simulink model "new24a"  (R2024a)
settings: Solver=FixedStepAuto  StartTime=0  StopTime=3  FixedStep=1e-6  RelTol=1e-3
InitFcn:
  | vdc=400
  | fsw=10000
  | Ld=0.393e-3
  | Lq=0.617e-3
  | R=0.0325
  | p=4
  | PM_flux=0.059
  | J=0.037
  | B=0.005
  | 
  | % Vehicle Model
  | Gr=1/5;                    %Gear Ratio
  | Trd=.508/2;                %Tire Radius
  | Drag= .25  ;               % Aro Dynamic Drag
  | Af= 2.23   ;               %Fontal Area
  | row= 1.225   ;             % Air Resistance
  | %Vm=260+140 ;              %Vehicle Weight
  | Vm=100;
  | Vw= Vm*9.81    ;           % Vehicle weight
  | Crr= .013  ;               %Rolling Coefficient
libraries: spsControlledVoltageSourceLib x1, slpidlib x1, spsPermanentMagnetSynchronousMachineLib x1, rllib x1, spsUniversalBridgeLib x1, spsabctodq0Lib x1, sps_lib x1
settings Model: Creator=lyche  LastModifiedBy=Saswata Mahato
settings SolverCC: ZeroCrossAlgorithm=Adaptive  AlgebraicLoopSolver=TrustRegion
settings DataIOCC: ReturnWorkspaceOutputs=off
settings OptimizationCC: ReuseModelBlockBuffer=off
settings DebuggingCC: MaxConsecutiveZCsMsg=none  UnconnectedInputMsg=warning  UnconnectedOutputMsg=warning  UnconnectedLineMsg=warning  ArithmeticOperatorsInVariantConditions=warning
settings ModelReferenceCC: EnableRefExpFcnMdlSchedulingChecks=on
settings SFSimCC: SimUseLocalCustomCode=off  CustomCodeUndefinedFunction=UseInterfaceOnly
settings RTWCC: RTWUseLocalCustomCode=off  GPUComputeCapability=3.5
settings CodeAppCC: StateflowObjectComments=on
settings SimscapeCC: SimscapeNormalizeSystem=off

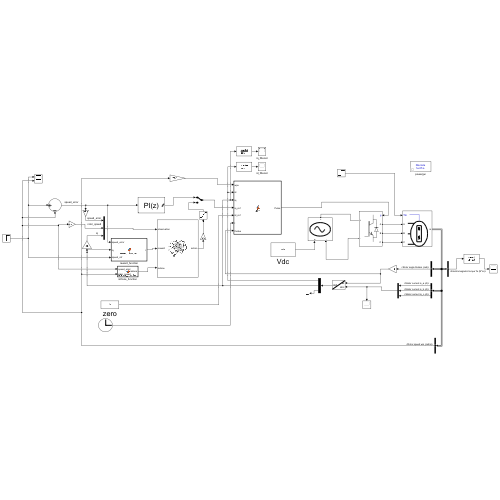
[thumbnail: Simulink's stored preview of the top-level diagram]
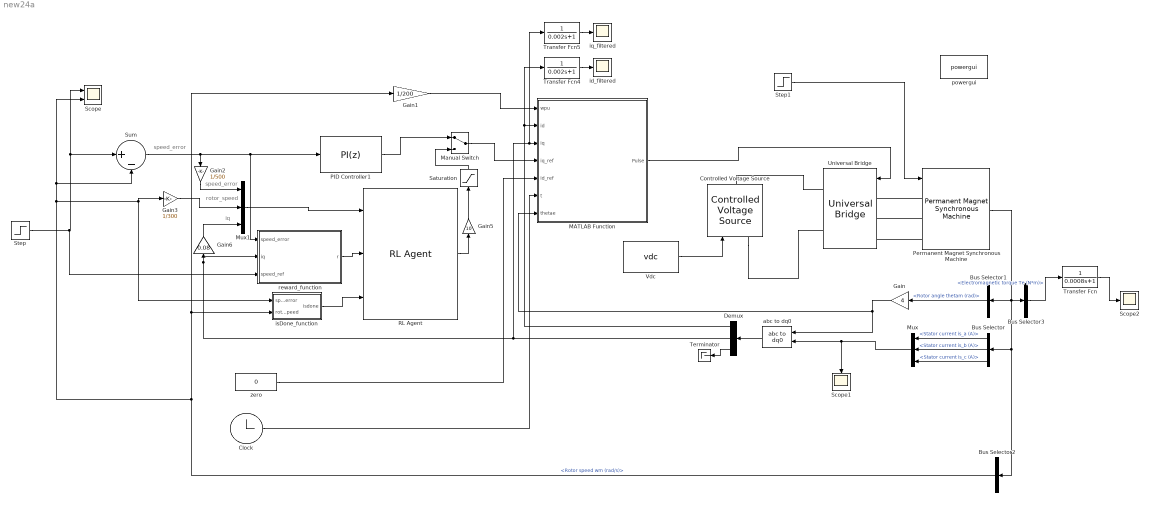
== system new24a ==
  note: iq
  note: rotor_speed
  note: speed_error
  note: speed_error
  Bus Selector : BusSelector  OutputSignals=Stator current is_a (A),Stator current is_b (A),Stator current is_c (A)
  Bus Selector1 : BusSelector  OutputSignals=Rotor angle thetam (rad)
  Bus Selector2 : BusSelector  OutputSignals=Rotor speed wm (rad/s)
  Bus Selector3 : BusSelector  OutputSignals=Electromagnetic torque Te (N*m)
  Clock : Clock
  Controlled Voltage Source : spsControlledVoltageSourceLib/Controlled Voltage Source  Initialize=off  Source_Type=AC  Amplitude=0  Phase=0  Frequency=0  Measurements=None
  Demux : Demux  Outputs=3
  Gain : Gain  Gain=4
  Gain1 : Gain  Gain=1/200
  Gain2 : Gain  Gain=1/500
  Gain3 : Gain  Gain=1/300
  Gain5 : Gain  Gain=10
  Gain6 : Gain  Gain=0.08
  MATLAB Function : MATLAB Function  TreatAsAtomicUnit=on
  Manual Switch : ManualSwitch
  Mux : Mux  Inputs=3
  Mux1 : Mux  Inputs=3
  PID Controller1 : slpidlib/PID Controller  Controller=PI  Form=Parallel  TimeDomain=Discrete-time  UseExternalTs=off  SampleTime=-1  IntegratorMethod=Forward Euler  FilterMethod=Forward Euler  ControllerParametersSource=internal  P=65.672  I=8.8746  UseKiTs=off  D=0  UseExternalDerivativeSource=off  N=100  UseFilter=on  TunerSelectOption=Transfer Function Based (PID Tuner App)  InitialConditionSource=internal  InitialConditionForIntegrator=0  InitialConditionForFilter=0  DifferentiatorICPrevScaledInput=0  ExternalReset=none  TrackingMode=off  Kt=1  LimitOutput=on  SatLimitsSource=internal  UpperSaturationLimit=500  LowerSaturationLimit=-500  LinearizeAsGain=off  AntiWindupMode=none  Kb=1  LimitIntegrator=off  UpperIntegratorSaturationLimit=inf  LowerIntegratorSaturationLimit=-inf  POutMin=[]  POutMax=[]  IOutMin=[]  IOutMax=[]  DOutMin=[]  DOutMax=[]  NOutMin=[]  NOutMax=[]  SumOutMin=[]  SumOutMax=[]  SaturationOutMin=[]  SaturationOutMax=[]  PParamMin=[]  PParamMax=[]  IParamMin=[]  IParamMax=[]  DParamMin=[]  DParamMax=[]  NParamMin=[]  NParamMax=[]  KbParamMin=[]  KbParamMax=[]  KtParamMin=[]  KtParamMax=[]  KbOutMin=[]  KbOutMax=[]  KtOutMin=[]  KtOutMax=[]  IntegratorOutMin=[]  IntegratorOutMax=[]  FilterOutMin=[]  FilterOutMax=[]  SumI1OutMin=[]  SumI1OutMax=[]  SumI2OutMin=[]  SumI2OutMax=[]  SumI3OutMin=[]  SumI3OutMax=[]  SumI4OutMin=[]  SumI4OutMax=[]  SumDOutMin=[]  SumDOutMax=[]  DifferentiatorOutMin=[]  DifferentiatorOutMax=[]  FilterDiffOutCoefMin=[]  FilterDiffOutCoefMax=[]  ReciprocalOutMin=[]  ReciprocalOutMax=[]  SumDenOutMin=[]  SumDenOutMax=[]  SumNumOutMin=[]  SumNumOutMax=[]  DivideOutMin=[]  DivideOutMax=[]  UdiffTsProdOutMin=[]  UdiffTsProdOutMax=[]  NTsProdOutMin=[]  NTsProdOutMax=[]  UintegralTsProdOutMin=[]  UintegralTsProdOutMax=[]  UngainTsProdOutMin=[]  UngainTsProdOutMax=[]  ClampingZeroOutDataTypeStr=Inherit: Inherit via back propagation  ClampingZeroOutMin=[]  ClampingZeroOutMax=[]  FilterDenConstantOutDataTypeStr=Inherit: Inherit via back propagation  FilterDenConstantOutMin=[]  FilterDenConstantOutMax=[]  PCopyOutDataTypeStr=Inherit: Inherit via back propagation  PCopyOutMin=[]  PCopyOutMax=[]  NCopyOutDataTypeStr=Inherit: Inherit via back propagation  NCopyOutMin=[]  NCopyOutMax=[]  IntegratorContinuousStateAttributes=''  IntegratorStateMustResolveToSignalObject=off  IntegratorRTWStateStorageClass=Auto  FilterContinuousStateAttributes=''  FilterStateMustResolveToSignalObject=off  FilterRTWStateStorageClass=Auto  ParallelPVariant=InternalParameters  IdealPVariant=Disabled  IVariant=InternalParameters  DVariant=Disabled  IntegratorVariant=Discrete  SatVariant=Enabled  AWVariant=Passthrough  PCopyVariant=Disabled  TRVariant=Disabled  FdbkBlocksVariant=Forward  IdealPFdbkVariant=Disabled  SatFdbkVariant=Disabled  DerivativeFilterVariant=Disabled  NVariant=Disabled  NCopyVariant=Disabled_SignalSpec  FilterICVariant=Disabled  IntegratorICVariant=InternalICs  ExternalResetVariant=Disabled  TRSumVariant=Passthrough  SumFdbkVariant=Disabled  SumVariant=Sum_PI  TsampFilterVariant=InternalTs  TsampNgainVariant=Passthrough  TsampIntegralVariant=Disabled_SignalSpec  ExternalSaturationOutDataTypeStr=Inherit: Same as second input  DerivativeSourceVariant=Disabled
  Permanent Magnet Synchronous Machine : spsPermanentMagnetSynchronousMachineLib/Permanent Magnet Synchronous Machine  NbPhases=3  FluxDistribution=Sinusoidal  RotorType=Salient-pole  MechanicalLoad=Torque Tm  PresetModel=No  ShowDetailedParameters=on  MeasurementBus=off  Resistance=0.0325  Inductance=8.5e-3  dqInductances=[0.393e-3,0.617e-3]  La=0.000395  MachineConstant=Flux linkage established by magnets (V.s)  Flux=0.059  VoltageCst=42.8057  TorqueCst=0.354  Flat=120  Mechanical=[0.037 0.005 4 0]  PolePairs=4  InitialConditions=[0,0, 0,0]  InitialConditions5ph=[0 0 0 0 0 0]  RefAngle=90 degrees behind phase A axis (modified Park)  IterativeDiscreteModel=Trapezoidal non iterative  TsBlock=-1  TsPowergui=0
  RL Agent : rllib/RL Agent  Agent=agent  ExternalActionAsInput=off  ProvideLastAction=off  ProvideCumRwd=off  TreatAsDirectFeedthrough=on  UseStrictObservationDataTypes=off
  Saturation : Saturate  UpperLimit=10  LowerLimit=-10
  Scope : Scope  NumInputPorts=2
  Scope1 : Scope
  Scope2 : Scope
  Step : Step  Time=0.5  Before=100  After=120  SampleTime=0
  Step1 : Step  Time=0.5  Before=20  After=70  SampleTime=0
  Sum : Sum  Inputs=|+-
  Terminator : Terminator
  Transfer Fcn : TransferFcn  Denominator=[0.0008 1]
  Transfer Fcn4 : TransferFcn  Denominator=[0.002 1]
  Transfer Fcn5 : TransferFcn  Denominator=[0.002 1]
  Universal Bridge : spsUniversalBridgeLib/Universal Bridge  Arms=3  SnubberResistance=1e5  SnubberCapacitance=inf  Device=IGBT / Diodes  Ron=1e-3  Lon=0  ForwardVoltages="[  0  0  ]"  ForwardVoltage=0  GTOparameters=[ 10e-6 , 20e-6 ]  IGBTparameters=[ 1e-6 , 2e-6 ]  Measurements=None  Measurements_2=None  converterType=Rectifier
  Vdc : Constant  Value=vdc
  abc to dq0 : spsabctodq0Lib/abc to dq0  Alignment=90 degrees behind phase A axis
  id_filtered : Scope
  iq_filtered : Scope
  "isDone_function " : MATLAB Function  TreatAsAtomicUnit=on
  powergui : sps_lib/powergui  Priority=1  SimulationMode=Discrete  SampleTime=10e-6  frequency=60  Iterations=50  frequencyindice=0  Pbase=100e6  ErrMax=1e-4  UnitsV=kV  UnitsW=MW  buscounter=0  FunctionMessages=off  echomessages=off  EnableUseOfTLC=off  CurrentSourceSwitches=off  DisableSnubberDevices=off  DisableRonSwitches=off  DisableVfSwitches=off  DisplayEquations=off  AutomaticDiscreteSolvers=off  SolverType=Tustin/Backward Euler (TBE)  Interpol=off  ExternalGateDelay=off  methode=off  Ts=100  x0status=blocks  SPID=on  SwTol=0  HookPort=off  NonlinearTolerance=1e-4  nMaxIteration=100  ContinueOnMaxIteration=off  RestoreLinks=warning  ResistiveCurrentMeasurement=off  Frange=[0:2:500]  Ylog=off  Xlog=on  ShowGrid=off  save=off  variable=ZData  structure=0  ZoomFFT=off  StartTime=0.0  cycles=1  DisplayStyle=1  fundamental=60  FreqAxis=off  MaxFrequency=1000  frequencyindicesteady=1  RmsSteady=1  display=off
  "reward_function " : MATLAB Function  TreatAsAtomicUnit=on
  zero : Constant  Value=0
  wires:
  Vdc/1 -> Controlled Voltage Source/1
  Clock/1 -> MATLAB Function/6(t)
  zero/1 -> MATLAB Function/5(id_ref)
  MATLAB Function/1(Pulse) -> Universal Bridge/1
  Permanent Magnet Synchronous Machine/1 -> Bus Selector3/1, Bus Selector1/1, Bus Selector/1, Bus Selector2/1
  Bus Selector1/1 -> Gain/1  "<Rotor angle thetam (rad)>"
  Gain/1 -> MATLAB Function/7(thetae), abc to dq0/2
  Bus Selector/1 -> Mux/1  "<Stator current is_a (A)>"
  Bus Selector/2 -> Mux/2  "<Stator current is_b (A)>"
  Bus Selector/3 -> Mux/3  "<Stator current is_c (A)>"
  Mux/1 -> Scope1/1, abc to dq0/1
  abc to dq0/1 -> Demux/1
  Demux/1 -> Transfer Fcn4/1, MATLAB Function/2(id)
  Demux/3 -> Terminator/1
  Bus Selector2/1 -> Gain1/1, "isDone_function "/2(rotor_speed), Sum/2, Scope/2, "isDone_function "/1(speed_error), Gain3/1  "<Rotor speed wm (rad/s)>"
  Gain1/1 -> MATLAB Function/1(wpu)
  Step1/1 -> Permanent Magnet Synchronous Machine/1
  Bus Selector3/1 -> Transfer Fcn/1  "<Electromagnetic torque Te (N*m)>"
  Transfer Fcn/1 -> Scope2/1
  Transfer Fcn4/1 -> id_filtered/1
  Transfer Fcn5/1 -> iq_filtered/1
  PID Controller1/1 -> Manual Switch/1
  RL Agent/1 -> Gain5/1
  "reward_function "/1(r) -> RL Agent/2
  Sum/1 -> "reward_function "/1(speed_error), PID Controller1/1, Gain2/1
  "isDone_function "/1(isdone) -> RL Agent/3
  Saturation/1 -> Manual Switch/2
  Gain2/1 -> Mux1/1
  Gain3/1 -> Mux1/2
  Gain5/1 -> Saturation/1
  Demux/2 -> Gain6/1, "reward_function "/2(iq), Transfer Fcn5/1, MATLAB Function/3(iq)
  Gain6/1 -> Mux1/3
  Mux1/1 -> RL Agent/1
  Step/1 -> "reward_function "/3(speed_ref), Sum/1, Scope/1
  Manual Switch/1 -> MATLAB Function/4(iq_ref)
  connections:
  Controlled Voltage Source/RConn1 -- Universal Bridge/RConn1
  Controlled Voltage Source/LConn1 -- Universal Bridge/RConn2
  Permanent Magnet Synchronous Machine/LConn2 -- Universal Bridge/LConn2
  Permanent Magnet Synchronous Machine/LConn3 -- Universal Bridge/LConn3
  Permanent Magnet Synchronous Machine/LConn1 -- Universal Bridge/LConn1

== matlab function new24a/reward_function  ==
  settings: updateMethod=DISCRETE  sampleTime=1e-3
  data: speed_error input; r output; iq input; speed_ref input
function r = reward_function(speed_error, iq, speed_ref)

normalized_error = abs(speed_error) / (abs(speed_ref) + 1);

% Main reward
r1 = exp(-5.0 * normalized_error^2);

% Reduced energy penalty
r2 = -0.00005 * iq^2;    % 10x smaller than before

% Bonus tiers
if normalized_error < 0.02
    bonus = 2.0;
elseif normalized_error < 0.05
    bonus = 0.5;
elseif normalized_error < 0.10
    bonus = 0.1;
else
    bonus = 0;
end

r = r1 + r2 + bonus;

end

== matlab function new24a/MATLAB Function ==
  settings: updateMethod=DISCRETE
  data: wpu input; id input; iq input; iq_ref input; id_ref input; t input; thetae input; Pulse output
function Pulse = MPC(wpu,id,iq,iq_ref,id_ref,t,thetae)

% Motor parameters
Ts   = 1e-5;
Ld   = 0.393e-3;
Lq   = 0.617e-3;
R    = 0.0325;
flux = 0.0590;
Vdc  = 400;
p    = 4;

% Electrical speed rad/s
we = wpu * 200 * (pi/30) * p;

% Clamp references
iq_ref = max(min(iq_ref, 10), -10);
id_ref = max(min(id_ref,  3),  -3);

% Use thetae DIRECTLY - do NOT add wpu*t (already integrated)
theta = -thetae;   % negate to match convention

% 8 switching vectors
S  = [0 0 0;
      1 0 0;
      1 1 0;
      0 1 0;
      0 1 1;
      0 0 1;
      1 0 1;
      1 1 1];

Sa = S(:,1); Sb = S(:,2); Sc = S(:,3);

% Phase voltages for all 8 vectors
Vinva = (Vdc*(2*Sa - Sb - Sc))/3;
Vinvb = (Vdc*(2*Sb - Sa - Sc))/3;
Vinvc = (Vdc*(2*Sc - Sb - Sa))/3;

% Standard Park transformation
% d-axis: cosine components
% q-axis: negative sine components
vsd = (2/3)*(Vinva.*cos(theta) ...
           + Vinvb.*cos(theta - 2*pi/3) ...
           + Vinvc.*cos(theta + 2*pi/3));

vsq = -(2/3)*(Vinva.*sin(theta) ...
            + Vinvb.*sin(theta - 2*pi/3) ...
            + Vinvc.*sin(theta + 2*pi/3));

% One-step PMSM prediction
id_p = id + Ts*((-R/Ld)*id + we*Lq*iq  + vsd/Ld);
iq_p = iq + Ts*((-R/Lq)*iq - we*(Ld*id + flux)/Lq + vsq/Lq);

% Cost function
err_id = id_ref - id_p;
err_iq = iq_ref - iq_p;

% Switching penalty
persistent S_prev;
if isempty(S_prev)
    S_prev = S(1,:);
end
sw_penalty = sum(abs(S - repmat(S_prev, size(S,1), 1)), 2);

cost = err_id.^2 + 2.0*err_iq.^2 + 0.001*sw_penalty;

% Select minimum cost vector
[~, idx] = min(cost);

% Gate signal LUT (top and bottom switches for A, B, C)
LUT = [0 1 0 1 0 1;
       1 0 0 1 0 1;
       1 0 1 0 0 1;
       0 1 1 0 0 1;
       0 1 1 0 1 0;
       0 1 0 1 1 0;
       1 0 0 1 1 0;
       1 0 1 0 1 0];

Pulse  = LUT(idx,:)';
S_prev = S(idx,:);

end

== matlab function new24a/isDone_function  ==
  settings: updateMethod=DISCRETE  sampleTime=1e-3
  data: speed_error input; isdone output; rotor_speed input
function isdone = isDone_function(speed_error, rotor_speed)

isdone = false;

% Kill episode if simulation is going unstable
if ~isfinite(speed_error) || ~isfinite(rotor_speed)
    isdone = true;
    return;
end

% Kill episode if speed error is catastrophically large
if abs(speed_error) > 300
    isdone = true;
    return;
end

% Kill episode if rotor speed physically impossible
if abs(rotor_speed) > 800
    isdone = true;
    return;
end

end
